simulink model "sema_imc"  (R2018b)
settings: Solver=VariableStepAuto  StartTime=0.0  StopTime=300  RelTol=1e-3
undefined symbols (not defined in the file or in its folder): a, b
libraries: simulink x1
settings Model: Creator=nahla  LastModifiedBy=nahla

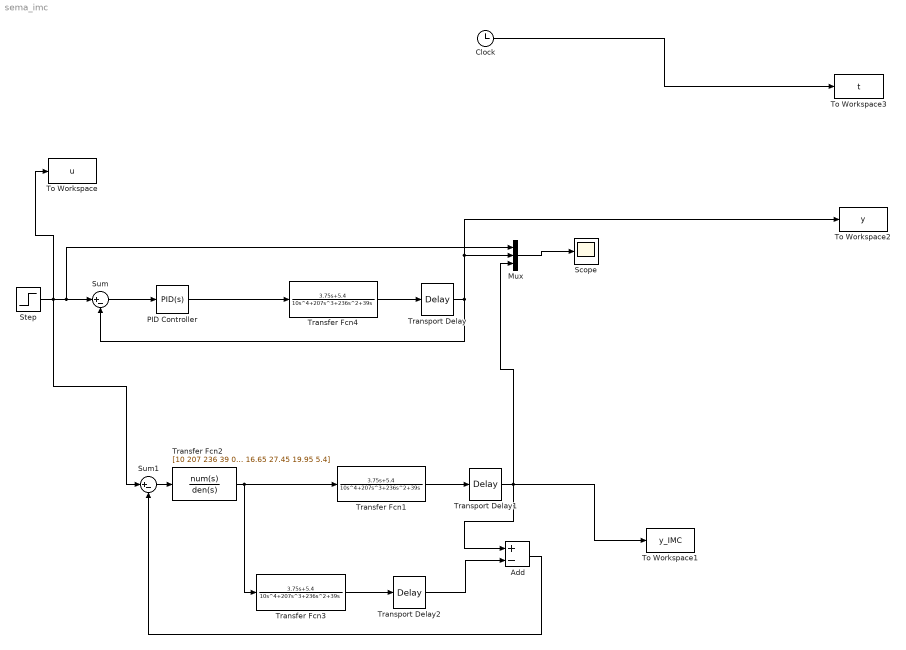
== system sema_imc ==
  Add : Sum  Inputs=+-
  Clock : Clock
  Mux : Mux  Inputs=3
  PID Controller : simulink/Continuous/PID Controller  Controller=PID  Form=Parallel  TimeDomain=Continuous-time  SampleTime=-1  IntegratorMethod=Forward Euler  FilterMethod=Forward Euler  ControllerParametersSource=internal  P=6.235  I=0  D=20.96  UseFilter=on  N=0  TunerSelectOption=Transfer Function Based (PID Tuner App)  InitialConditionSource=internal  InitialConditionForIntegrator=0  InitialConditionForFilter=0  DifferentiatorICPrevScaledInput=0  ExternalReset=none  TrackingMode=off  Kt=1  LimitOutput=off  UpperSaturationLimit=inf  LowerSaturationLimit=-inf  LinearizeAsGain=on  AntiWindupMode=none  Kb=1  POutMin=[]  POutMax=[]  IOutMin=[]  IOutMax=[]  DOutMin=[]  DOutMax=[]  NOutMin=[]  NOutMax=[]  SumOutMin=[]  SumOutMax=[]  SaturationOutMin=[]  SaturationOutMax=[]  PParamMin=[]  PParamMax=[]  IParamMin=[]  IParamMax=[]  DParamMin=[]  DParamMax=[]  NParamMin=[]  NParamMax=[]  KbParamMin=[]  KbParamMax=[]  KtParamMin=[]  KtParamMax=[]  KbOutMin=[]  KbOutMax=[]  KtOutMin=[]  KtOutMax=[]  IntegratorOutMin=[]  IntegratorOutMax=[]  FilterOutMin=[]  FilterOutMax=[]  SumI1OutMin=[]  SumI1OutMax=[]  SumI2OutMin=[]  SumI2OutMax=[]  SumI3OutMin=[]  SumI3OutMax=[]  SumI4OutMin=[]  SumI4OutMax=[]  SumDOutMin=[]  SumDOutMax=[]  DifferentiatorOutMin=[]  DifferentiatorOutMax=[]  FilterDiffOutCoefMin=[]  FilterDiffOutCoefMax=[]  ReciprocalOutMin=[]  ReciprocalOutMax=[]  SumDenOutMin=[]  SumDenOutMax=[]  SumNumOutMin=[]  SumNumOutMax=[]  DivideOutMin=[]  DivideOutMax=[]  IntegratorContinuousStateAttributes=''  IntegratorStateMustResolveToSignalObject=off  IntegratorRTWStateStorageClass=Auto  FilterContinuousStateAttributes=''  FilterStateMustResolveToSignalObject=off  FilterRTWStateStorageClass=Auto  ParallelPVariant=InternalParameters  IdealPVariant=Disabled  IVariant=InternalParameters  DVariant=InternalParameters  IntegratorVariant=Continuous  SatVariant=Disabled  AWVariant=Passthrough  PCopyVariant=Disabled  TRVariant=Disabled  FdbkBlocksVariant=Forward  IdealPFdbkVariant=Disabled  SatFdbkVariant=Disabled  DerivativeFilterVariant=ContFilter  NVariant=InternalParameters  NCopyVariant=Disabled  FilterICVariant=InternalICsFilter  IntegratorICVariant=InternalICs  ExternalResetVariant=Disabled  TRSumVariant=Passthrough  SumFdbkVariant=Disabled  SumVariant=Sum_PID
  Scope : Scope
  Step : Step  SampleTime=0
  Sum : Sum  Inputs=|+-
  Sum1 : Sum  Inputs=|+-
  To Workspace : ToWorkspace  VariableName=u  SampleTime=-1
  To Workspace1 : ToWorkspace  VariableName=y_IMC  SampleTime=-1
  To Workspace2 : ToWorkspace  VariableName=y  SampleTime=-1
  To Workspace3 : ToWorkspace  VariableName=t  SampleTime=-1
  Transfer Fcn1 : TransferFcn  Numerator=[3.75 5.4]  Denominator="[10 207 236  39 0]"
  Transfer Fcn2 : TransferFcn  Numerator=[10 207 236 39 0]  Denominator=[3.75 16.65 27.45 19.95 5.4]
  Transfer Fcn3 : TransferFcn  Numerator=[3.75 5.4]  Denominator="[10 207 236  39 0]"
  Transfer Fcn4 : TransferFcn  Numerator=[3.75 5.4]  Denominator="[10 207 236  39 0]"
  Transport Delay : TransportDelay  DelayTime=a+b+10
  Transport Delay1 : TransportDelay  DelayTime=a+b+10
  Transport Delay2 : TransportDelay  DelayTime=a+b+10
  wires:
  Add/1 -> Sum1/2
  Clock/1 -> To Workspace3/1
  Transport Delay2/1 -> Add/2
  Transport Delay1/1 -> To Workspace1/1, Add/1, Mux/3
  Transfer Fcn2/1 -> Transfer Fcn3/1, Transfer Fcn1/1
  Transport Delay/1 -> Sum/2, Mux/2, To Workspace2/1
  Step/1 -> To Workspace/1, Sum1/1, Mux/1, Sum/1
  Mux/1 -> Scope/1
  Sum1/1 -> Transfer Fcn2/1
  PID Controller/1 -> Transfer Fcn4/1
  Sum/1 -> PID Controller/1
  Transfer Fcn4/1 -> Transport Delay/1
  Transfer Fcn1/1 -> Transport Delay1/1
  Transfer Fcn3/1 -> Transport Delay2/1
